simulink model "motor_no_feedforward_LSF_Kvi"  (R2024a)
settings: Solver=VariableStepAuto  StartTime=0.0  StopTime=total_time  FixedStep=0.001  MaxStep=sampT  RelTol=1e-3
values from neighbouring files (symbols this model uses):
  B_sys = 0.0003457395    [check_simulation_no_feedforward_v14.m]
  BW_Current = 2000    [check_simulation_no_feedforward_v14.m]
  C12 = 0.03844    [check_simulation_no_feedforward_v14.m]
  close_friction = 1    [check_simulation_no_feedforward_v14.m]    (also in simulation_no_feedforward_step.m; simulation_no_feedforward_step_sat.m; simulation_no_feedforward_step_sat_enable.m; simulation_no_feedforward_trap.m)
  close_position = 1    [check_simulation_no_feedforward_v14.m]    (also in simulation_no_feedforward_step.m; simulation_no_feedforward_step_sat.m; simulation_no_feedforward_step_sat_enable.m; simulation_no_feedforward_trap.m)
  close_velocity = 1    [check_simulation_no_feedforward_v14.m]    (also in simulation_no_feedforward_step.m; simulation_no_feedforward_step_sat.m; simulation_no_feedforward_step_sat_enable.m; simulation_no_feedforward_trap.m)
  fc = [-0.033249, 0.027123]    [check_simulation_no_feedforward_v14.m]
  fs = [-0.04, 0.04]    [check_simulation_no_feedforward_v14.m]
  J = J1 + J2    (= 0.000116959)    [check_simulation_no_feedforward_v14.m]
  J1 = 45e-6    (= 4.5e-05)    [check_simulation_no_feedforward_v14.m]
  J2 = 71.959e-6    (= 7.1959e-05)    [check_simulation_no_feedforward_v14.m]
  K12 = 1830.016    [check_simulation_no_feedforward_v14.m]
  Kpp = 400.0    (= 400)    [check_simulation_no_feedforward_v14.m]
  Kvp = 400.0    (= 400)    [check_simulation_no_feedforward_v14.m]
  sampT = 0.001    [check_simulation_no_feedforward_v14.m]
  start_position = 0.0    (= 0)    [check_simulation_no_feedforward_v14.m]
  v_fric = 0.0    (= 0)    [check_simulation_no_feedforward_v14.m]
undefined symbols (not defined in the file or in its folder): DiscIntNeverNeededParam, Kvi
settings Model: Creator=ricky  LastModifiedBy=VSCLAB-3060
settings DataIOCC: SaveOutput=off  SignalLogging=off  DSMLogging=off  ReturnWorkspaceOutputs=off

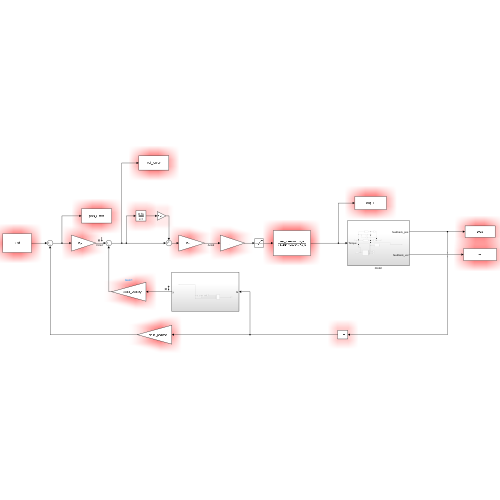
[thumbnail: Simulink's stored preview of the top-level diagram]
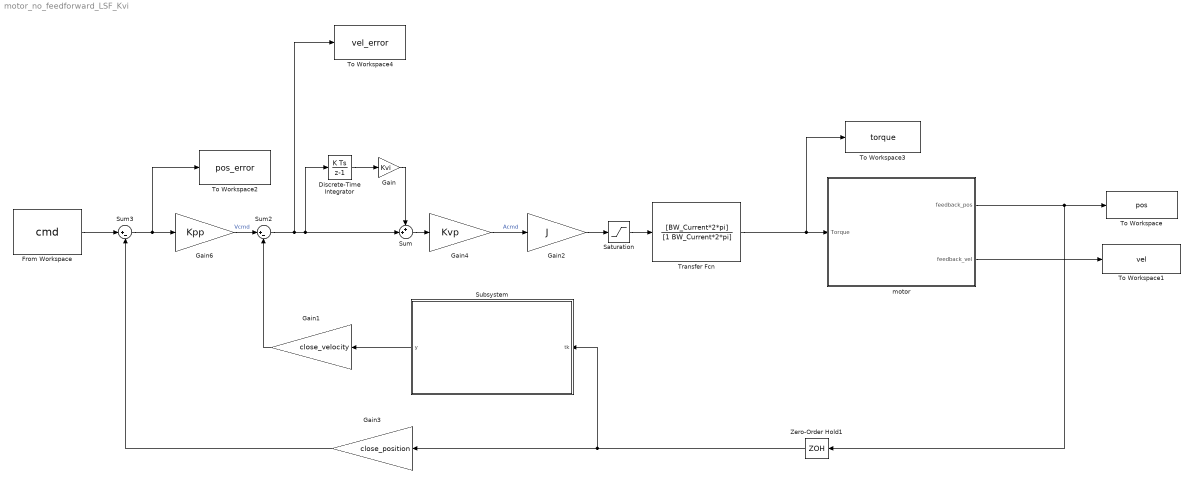
== system motor_no_feedforward_LSF_Kvi ==
  Discrete-Time Integrator : DiscreteIntegrator  SampleTime=sampT  ICPrevOutput=DiscIntNeverNeededParam  ICPrevScaledInput=DiscIntNeverNeededParam
  From Workspace : FromWorkspace  VariableName=cmd  SampleTime=sampT
  Gain : Gain  Gain=Kvi
  Gain1 : Gain  Gain=close_velocity
  Gain2 : Gain  Gain=J
  Gain3 : Gain  Gain=close_position
  Gain4 : Gain  Gain=Kvp
  Gain6 : Gain  Gain=Kpp
  Saturation : Saturate  UpperLimit=4.45  LowerLimit=-4.45
  Subsystem : Subsystem
  Sum : Sum  Inputs=++|
  Sum2 : Sum  Inputs=|+-
  Sum3 : Sum  Inputs=|+-
  To Workspace : ToWorkspace  VariableName=pos  SampleTime=sampT
  To Workspace1 : ToWorkspace  VariableName=vel  SampleTime=sampT
  To Workspace2 : ToWorkspace  VariableName=pos_error  SampleTime=sampT
  To Workspace3 : ToWorkspace  VariableName=torque  SampleTime=sampT
  To Workspace4 : ToWorkspace  VariableName=vel_error  SampleTime=sampT
  Transfer Fcn : TransferFcn  Numerator=[BW_Current*2*pi]  Denominator=[1 BW_Current*2*pi]
  Zero-Order Hold1 : ZeroOrderHold  SampleTime=sampT
  motor : Subsystem
  wires:
  motor/2(feedback_vel) -> To Workspace1/1
  Gain4/1 -> Gain2/1  "Acmd"
  Sum3/1 -> To Workspace2/1, Gain6/1
  From Workspace/1 -> Sum3/1
  Sum2/1 -> To Workspace4/1, Sum/2, Discrete-Time Integrator/1
  Gain6/1 -> Sum2/1  "Vcmd"
  Gain2/1 -> Saturation/1
  Zero-Order Hold1/1 -> Subsystem/1(tk), Gain3/1
  motor/1(feedback_pos) -> Zero-Order Hold1/1, To Workspace/1
  Transfer Fcn/1 -> To Workspace3/1, motor/1(Torque)
  Saturation/1 -> Transfer Fcn/1
  Discrete-Time Integrator/1 -> Gain/1
  Sum/1 -> Gain4/1
  Gain/1 -> Sum/1
  Subsystem/1(y) -> Gain1/1
  Gain1/1 -> Sum2/2
  Gain3/1 -> Sum3/2

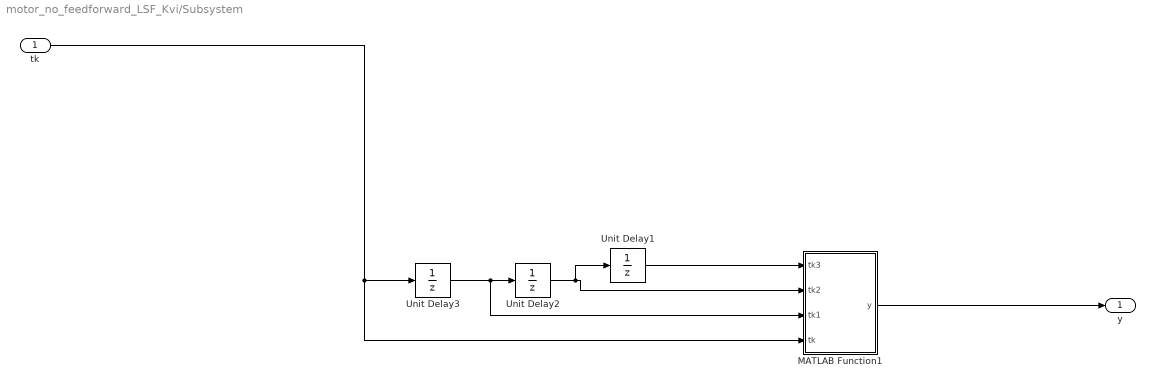
== system motor_no_feedforward_LSF_Kvi/Subsystem ==
  tk : Inport
  MATLAB Function1 : MATLAB Function  TreatAsAtomicUnit=on
  Unit Delay1 : UnitDelay  InitialCondition=start_position  SampleTime=sampT  HasFrameUpgradeWarning=on
  Unit Delay2 : UnitDelay  InitialCondition=start_position  SampleTime=sampT  HasFrameUpgradeWarning=on
  Unit Delay3 : UnitDelay  InitialCondition=start_position  SampleTime=sampT  HasFrameUpgradeWarning=on
  y : Outport
  wires:
  tk/1 -> MATLAB Function1/4(tk), Unit Delay3/1
  Unit Delay3/1 -> MATLAB Function1/3(tk1), Unit Delay2/1
  Unit Delay2/1 -> MATLAB Function1/2(tk2), Unit Delay1/1
  MATLAB Function1/1(y) -> y/1
  Unit Delay1/1 -> MATLAB Function1/1(tk3)

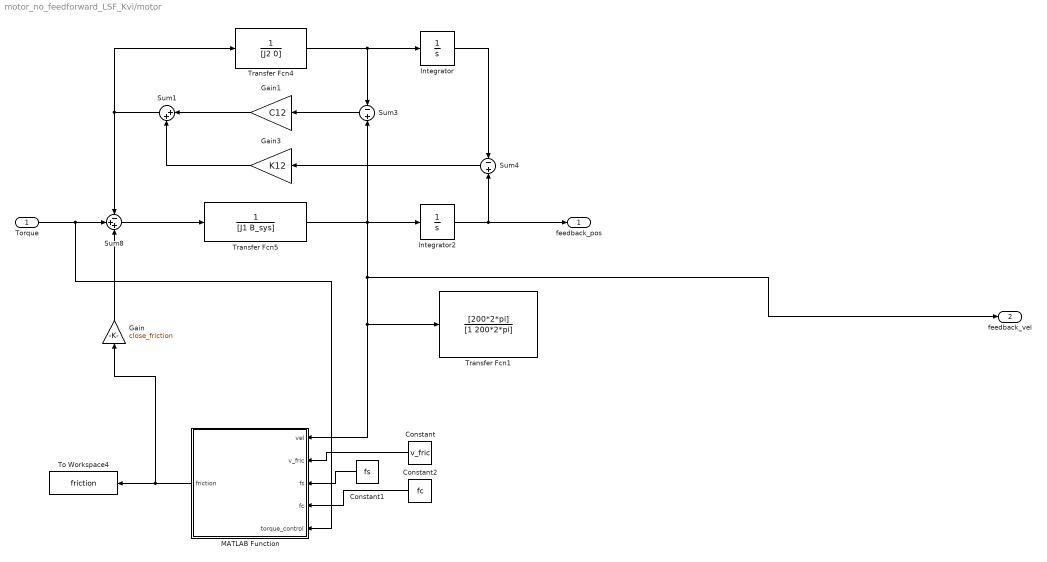
== system motor_no_feedforward_LSF_Kvi/motor ==
  Torque : Inport
  Constant : Constant  Value=v_fric
  Constant1 : Constant  Value=fs
  Constant2 : Constant  Value=fc
  Gain : Gain  Gain=close_friction
  Gain1 : Gain  Gain=C12
  Gain3 : Gain  Gain=K12
  Integrator : Integrator  InitialCondition=start_position
  Integrator2 : Integrator  InitialCondition=start_position
  MATLAB Function : MATLAB Function  TreatAsAtomicUnit=on
  Sum1 : Sum  Inputs=|++
  Sum3 : Sum  Inputs=-|+
  Sum4 : Sum  Inputs=-|+
  Sum8 : Sum  Inputs=-++
  To Workspace4 : ToWorkspace  VariableName=friction  SampleTime=sampT
  Transfer Fcn1 : TransferFcn  Numerator=[200*2*pi]  Denominator=[1 200*2*pi]
  Transfer Fcn4 : TransferFcn  Denominator=[J2 0]
  Transfer Fcn5 : TransferFcn  Denominator=[J1 B_sys]
  feedback_pos : Outport
  feedback_vel : Outport  Port=2
  wires:
  Gain1/1 -> Sum1/1
  Sum4/1 -> Gain3/1
  Transfer Fcn4/1 -> Sum3/1, Integrator/1
  Sum3/1 -> Gain1/1
  Sum8/1 -> Transfer Fcn5/1
  Gain3/1 -> Sum1/2
  Sum1/1 -> Transfer Fcn4/1, Sum8/1
  Integrator/1 -> Sum4/1
  Integrator2/1 -> Sum4/2, feedback_pos/1
  Transfer Fcn5/1 -> Sum3/2, feedback_vel/1, Transfer Fcn1/1, MATLAB Function/1(vel), Integrator2/1
  MATLAB Function/1(friction) -> Gain/1, To Workspace4/1
  Constant1/1 -> MATLAB Function/3(fs)
  Torque/1 -> MATLAB Function/5(torque_control), Sum8/2
  Constant/1 -> MATLAB Function/2(v_fric)
  Constant2/1 -> MATLAB Function/4(fc)
  Gain/1 -> Sum8/3

== matlab function motor_no_feedforward_LSF_Kvi/Subsystem/MATLAB Function1 ==
  data: tk3 input; y output; tk2 input; tk1 input; tk input
function y = fcn(tk3, tk2, tk1, tk)

y = (-0.3*tk3 - 0.1*tk2 + 0.1*tk1 + 0.3*tk)/0.001;

== matlab function motor_no_feedforward_LSF_Kvi/motor/MATLAB Function ==
  data: vel input; friction output; v_fric input; fs input; fc input; torque_control input
function friction = fcn(vel, v_fric, fs, fc, torque_control)
    % Initialize friction
    friction = 0;
    
    % Coulomb Friction: If velocity exceeds threshold
    if vel > v_fric
        friction = fc(2);
    elseif vel < -v_fric
        friction = fc(1);
        
    % Static Friction: If velocity is small (near zero)
    elseif abs(vel) <= v_fric
        if torque_control > 0 && torque_control < fs(2)
            friction = torque_control;
        elseif torque_control < 0 && torque_control > fs(1)
            friction = torque_control;
        elseif torque_control >= fs(2)
            friction = fs(2);
        elseif torque_control <= fs(1)
            friction = fs(1);
        end
    end
end
